simulink model "Powertrain"  (R2018b)
settings: configuration reference "Physics" (kept outside this file)
model workspace (MAT data in the model file):
  m = 1000
undefined symbols (not defined in the file): POWTR__CLUTCH__clutch_time_s, POWTR__CLUTCH__T_max_cap_Nm, POWTR__DIFFERENTIAL__c_diff_efficiency, POWTR__DIFFERENTIAL__c_diff_ratio, POWTR__DIFFERENTIAL__f_diff_efficiency, POWTR__DIFFERENTIAL__f_diff_ratio, POWTR__DIFFERENTIAL__I_drivetrain_kgm2, POWTR__DIFFERENTIAL__r_diff_efficiency, POWTR__DIFFERENTIAL__r_diff_ratio, POWTR__ENGINE__I_engine_kgm2, POWTR__ENGINE__n_0_rpm, POWTR__ENGINE__n_idle_rpm, POWTR__ENGINE__n_lb_rpm__1, POWTR__ENGINE__n_lb_rpm__2, POWTR__ENGINE__n_lb_rpm__3, POWTR__ENGINE__n_lb_rpm__4, POWTR__ENGINE__n_lb_rpm__5, POWTR__ENGINE__n_lb_rpm__6, POWTR__ENGINE__n_lb_rpm__7, POWTR__ENGINE__n_limit_rpm, POWTR__ENGINE__n_ub_rpm, POWTR__LAYOUT__p_torque_rear, POWTR__MODE__activate_CombustionEngine, POWTR__MODE__activate_ManualGearbox, POWTR__MODE__activate_ThrottleInterface, POWTR__TRANSMISSION__gear__1, POWTR__TRANSMISSION__gear__2, POWTR__TRANSMISSION__gear__3, POWTR__TRANSMISSION__gear__4, POWTR__TRANSMISSION__gear__5, POWTR__TRANSMISSION__gear__6, POWTR__TRANSMISSION__gear__7, POWTR__TRANSMISSION__gear_efficiency__1, POWTR__TRANSMISSION__gear_efficiency__2, POWTR__TRANSMISSION__gear_efficiency__3, POWTR__TRANSMISSION__gear_efficiency__4, POWTR__TRANSMISSION__gear_efficiency__5, POWTR__TRANSMISSION__gear_efficiency__6, POWTR__TRANSMISSION__gear_efficiency__7, POWTR__TRANSMISSION__gear_ratio__1, POWTR__TRANSMISSION__gear_ratio__2, POWTR__TRANSMISSION__gear_ratio__3, POWTR__TRANSMISSION__gear_ratio__4, POWTR__TRANSMISSION__gear_ratio__5, POWTR__TRANSMISSION__gear_ratio__6, POWTR__TRANSMISSION__gear_ratio__7, POWTR__TRANSMISSION__I_transmission_kgm2, tireFL__MFSIMPLE__r_tire_m, tireFR__MFSIMPLE__r_tire_m, tireRL__MFSIMPLE__r_tire_m, tireRR__MFSIMPLE__r_tire_m, VEH__VehicleData__l_WheelbaseF_m, VEH__VehicleData__l_WheelbaseTotal_m, VEH__VehicleData__w_TrackF_m, VEH__VehicleData__w_TrackR_m
libraries: simulink x4
settings Model: DataDictionary=vehicleparameters_vehdynsim.sldd  PauseTimes=9.280  Creator=wischnewski  LastModifiedBy=ga25xiw

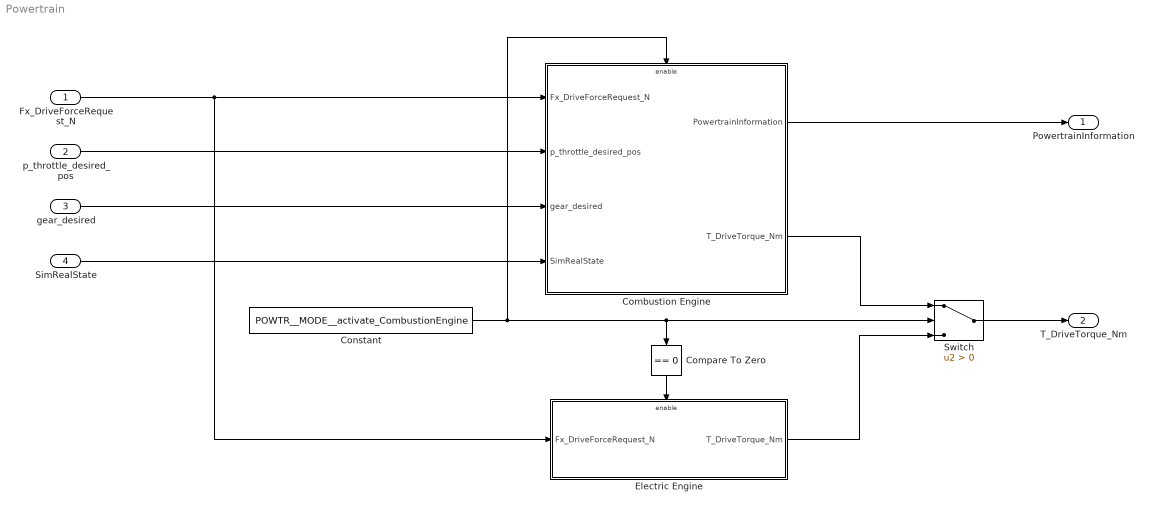
== system Powertrain ==
  Fx_DriveForceRequest_N : Inport
  p_throttle_desired_pos : Inport  Port=2
  gear_desired : Inport  Port=3
  SimRealState : Inport  Port=4  OutDataTypeStr=Bus: SimRealState
  Combustion Engine : Subsystem  TreatAsAtomicUnit=on
  Compare To Zero : simulink/Logic and Bit Operations/Compare To Zero  relop===  OutDataTypeStr=boolean
  Constant : Constant  Value=POWTR__MODE__activate_CombustionEngine
  Electric Engine : Subsystem  TreatAsAtomicUnit=on
  Switch : Switch  Criteria=u2 > Threshold
  PowertrainInformation : Outport  OutDataTypeStr=Bus: PowertrainInformation
  T_DriveTorque_Nm : Outport  Port=2
  wires:
  Constant/1 -> Combustion Engine/Enable, Switch/2, Compare To Zero/1
  gear_desired/1 -> Combustion Engine/3(gear_desired)
  Fx_DriveForceRequest_N/1 -> Electric Engine/1(Fx_DriveForceRequest_N), Combustion Engine/1(Fx_DriveForceRequest_N)
  Switch/1 -> T_DriveTorque_Nm/1
  Combustion Engine/2(T_DriveTorque_Nm) -> Switch/1
  Compare To Zero/1 -> Electric Engine/Enable
  p_throttle_desired_pos/1 -> Combustion Engine/2(p_throttle_desired_pos)
  Electric Engine/1(T_DriveTorque_Nm) -> Switch/3
  SimRealState/1 -> Combustion Engine/4(SimRealState)
  Combustion Engine/1(PowertrainInformation) -> PowertrainInformation/1

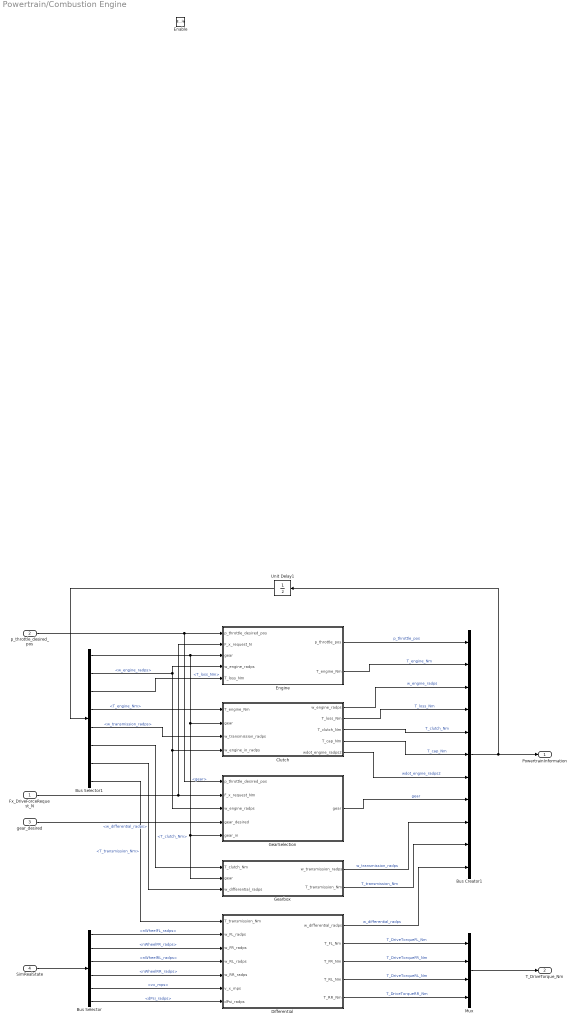
== system Powertrain/Combustion Engine ==
  Fx_DriveForceRequest_N : Inport
  p_throttle_desired_pos : Inport  Port=2
  gear_desired : Inport  Port=3
  SimRealState : Inport  Port=4  OutDataTypeStr=Bus: SimRealState
  Enable : EnablePort
  Bus Creator1 : BusCreator  Inputs=11  OutDataTypeStr=Bus: PowertrainInformation
  Bus Selector : BusSelector  OutputSignals=nWheelFL_radps,nWheelFR_radps,nWheelRL_radps,nWheelRR_radps,vx_mps,dPsi_radps
  Bus Selector1 : BusSelector  OutputSignals=gear,w_engine_radps,T_loss_Nm,T_engine_Nm,w_transmission_radps,T_clutch_Nm,w_differential_radps,T_transmission_Nm
  Clutch : Subsystem
  Differential : Subsystem
  Engine : Subsystem
  GearSelection : Subsystem
  Gearbox : Subsystem
  Mux : Mux
  Unit Delay1 : UnitDelay  SampleTime=-1
  PowertrainInformation : Outport  OutDataTypeStr=Bus: PowertrainInformation
  T_DriveTorque_Nm : Outport  Port=2
  wires:
  Differential/1(w_differential_radps) -> Bus Creator1/11  "w_differential_radps"
  Differential/4(T_RL_Nm) -> Mux/3  "T_DriveTorqueRL_Nm"
  Bus Selector1/5 -> Clutch/3(w_transmission_radps)  "<w_transmission_radps>"
  p_throttle_desired_pos/1 -> GearSelection/1(p_throttle_desired_pos), Engine/1(p_throttle_desired_pos)
  Differential/5(T_RR_Nm) -> Mux/4  "T_DriveTorqueRR_Nm"
  Engine/1(p_throttle_pos) -> Bus Creator1/1  "p_throttle_pos"
  Clutch/1(w_engine_radps) -> Bus Creator1/3  "w_engine_radps"
  Bus Creator1/1 -> Unit Delay1/1, PowertrainInformation/1
  Gearbox/1(w_transmission_radps) -> Bus Creator1/9  "w_transmission_radps"
  Mux/1 -> T_DriveTorque_Nm/1
  Bus Selector/1 -> Differential/2(w_FL_radps)  "<nWheelFL_radps>"
  Clutch/2(T_loss_Nm) -> Bus Creator1/4  "T_loss_Nm"
  Engine/2(T_engine_Nm) -> Bus Creator1/2  "T_engine_Nm"
  Fx_DriveForceRequest_N/1 -> Engine/2(F_x_request_N), GearSelection/2(F_x_request_Nm)
  Bus Selector/6 -> Differential/7(dPsi_radps)  "<dPsi_radps>"
  GearSelection/1(gear) -> Bus Creator1/8  "gear"
  Bus Selector/4 -> Differential/5(w_RR_radps)  "<nWheelRR_radps>"
  Gearbox/2(T_transmission_Nm) -> Bus Creator1/10  "T_transmission_Nm"
  SimRealState/1 -> Bus Selector/1
  Differential/2(T_FL_Nm) -> Mux/1  "T_DriveTorqueFL_Nm"
  Bus Selector/5 -> Differential/6(v_x_mps)  "<vx_mps>"
  Bus Selector1/6 -> Gearbox/1(T_clutch_Nm)  "<T_clutch_Nm>"
  Bus Selector/3 -> Differential/4(w_RL_radps)  "<nWheelRL_radps>"
  gear_desired/1 -> GearSelection/4(gear_desired)
  Differential/3(T_FR_Nm) -> Mux/2  "T_DriveTorqueFR_Nm"
  Clutch/3(T_clutch_Nm) -> Bus Creator1/5  "T_clutch_Nm"
  Bus Selector1/4 -> Clutch/1(T_engine_Nm)  "<T_engine_Nm>"
  Bus Selector1/2 -> Engine/4(w_engine_radps), GearSelection/3(w_engine_radps), Clutch/4(w_engine_in_radps)  "<w_engine_radps>"
  Bus Selector/2 -> Differential/3(w_FR_radps)  "<nWheelFR_radps>"
  Bus Selector1/7 -> Gearbox/3(w_differential_radps)  "<w_differential_radps>"
  Clutch/4(T_cap_Nm) -> Bus Creator1/6  "T_cap_Nm"
  Clutch/5(wdot_engine_radps2) -> Bus Creator1/7  "wdot_engine_radps2"
  Bus Selector1/3 -> Engine/5(T_loss_Nm)  "<T_loss_Nm>"
  Bus Selector1/1 -> Engine/3(gear), Gearbox/2(gear), GearSelection/5(gear_in), Clutch/2(gear)  "<gear>"
  Bus Selector1/8 -> Differential/1(T_transmission_Nm)  "<T_transmission_Nm>"
  Unit Delay1/1 -> Bus Selector1/1

== system Powertrain/Electric Engine ==
  Fx_DriveForceRequest_N : Inport
  Enable : EnablePort
  Constant : Constant  Value=POWTR__LAYOUT__p_torque_rear
  Demux : Demux
  EelctricEngine : MATLAB Function  TreatAsAtomicUnit=on
  Gain4 : Gain  Gain=tireFL__MFSIMPLE__r_tire_m
  Gain5 : Gain  Gain=tireFR__MFSIMPLE__r_tire_m
  Gain6 : Gain  Gain=tireRL__MFSIMPLE__r_tire_m
  Gain7 : Gain  Gain=tireRR__MFSIMPLE__r_tire_m
  Mux : Mux
  Saturation : Saturate  UpperLimit=inf  LowerLimit=0
  Transfer Fcn : TransferFcn  Denominator=[0.02 1]
  T_DriveTorque_Nm : Outport
  wires:
  EelctricEngine/1(F_DriveForce_N) -> Demux/1
  Demux/1 -> Gain4/1
  Gain6/1 -> Mux/3  "T_DriveTorqueRL_Nm"
  Constant/1 -> EelctricEngine/2(p_torque_rear)
  Saturation/1 -> Transfer Fcn/1
  Demux/3 -> Gain6/1
  Demux/2 -> Gain5/1
  Gain5/1 -> Mux/2  "T_DriveTorqueFR_Nm"
  Gain4/1 -> Mux/1  "T_DriveTorqueFL_Nm"
  Transfer Fcn/1 -> EelctricEngine/1(F_x_request_N)
  Fx_DriveForceRequest_N/1 -> Saturation/1
  Gain7/1 -> Mux/4  "T_DriveTorqueRR_Nm"
  Demux/4 -> Gain7/1
  Mux/1 -> T_DriveTorque_Nm/1

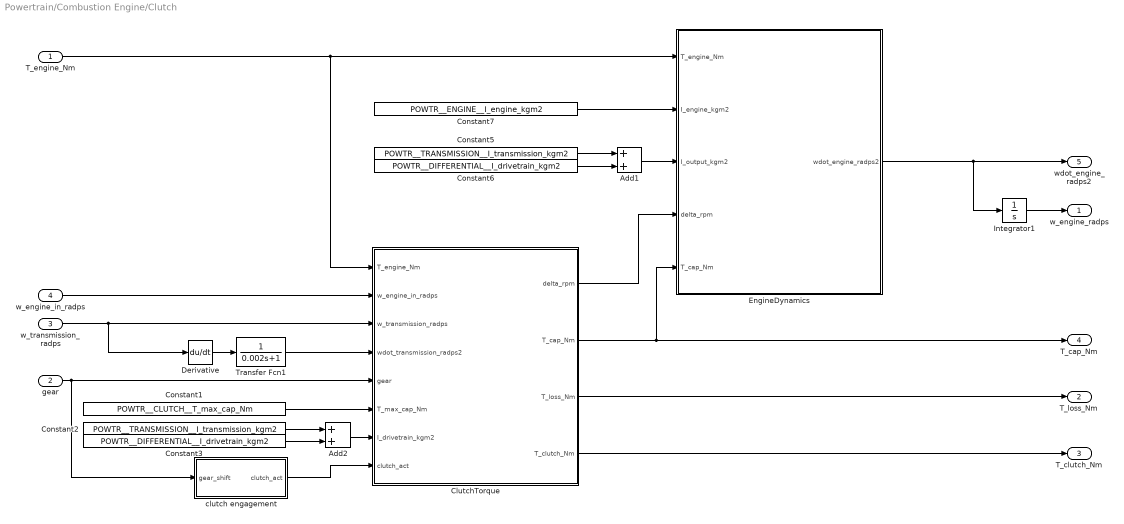
== system Powertrain/Combustion Engine/Clutch ==
  T_engine_Nm : Inport
  gear : Inport  Port=2
  w_transmission_radps : Inport  Port=3
  w_engine_in_radps : Inport  Port=4
  Add1 : Sum
  Add2 : Sum
  ClutchTorque : MATLAB Function  TreatAsAtomicUnit=on
  Constant1 : Constant  Value=POWTR__CLUTCH__T_max_cap_Nm
  Constant2 : Constant  Value=POWTR__TRANSMISSION__I_transmission_kgm2
  Constant3 : Constant  Value=POWTR__DIFFERENTIAL__I_drivetrain_kgm2
  Constant5 : Constant  Value=POWTR__TRANSMISSION__I_transmission_kgm2
  Constant6 : Constant  Value=POWTR__DIFFERENTIAL__I_drivetrain_kgm2
  Constant7 : Constant  Value=POWTR__ENGINE__I_engine_kgm2
  Derivative : Derivative
  EngineDynamics : MATLAB Function  TreatAsAtomicUnit=on
  Integrator1 : Integrator  InitialCondition=POWTR__ENGINE__n_0_rpm * ((2*pi)/60)
  Transfer Fcn1 : TransferFcn  Denominator=[0.002 1]
  clutch engagement : Subsystem
  w_engine_radps : Outport
  T_loss_Nm : Outport  Port=2
  T_clutch_Nm : Outport  Port=3
  T_cap_Nm : Outport  Port=4
  wdot_engine_radps2 : Outport  Port=5
  wires:
  ClutchTorque/1(delta_rpm) -> EngineDynamics/4(delta_rpm)
  clutch engagement/1(clutch_act) -> ClutchTorque/8(clutch_act)
  Integrator1/1 -> w_engine_radps/1
  w_transmission_radps/1 -> Derivative/1, ClutchTorque/3(w_transmission_radps)
  ClutchTorque/3(T_loss_Nm) -> T_loss_Nm/1
  ClutchTorque/2(T_cap_Nm) -> T_cap_Nm/1, EngineDynamics/5(T_cap_Nm)
  Constant7/1 -> EngineDynamics/2(I_engine_kgm2)
  ClutchTorque/4(T_clutch_Nm) -> T_clutch_Nm/1
  w_engine_in_radps/1 -> ClutchTorque/2(w_engine_in_radps)
  T_engine_Nm/1 -> ClutchTorque/1(T_engine_Nm), EngineDynamics/1(T_engine_Nm)
  Constant1/1 -> ClutchTorque/6(T_max_cap_Nm)
  Add2/1 -> ClutchTorque/7(I_drivetrain_kgm2)
  Add1/1 -> EngineDynamics/3(I_output_kgm2)
  gear/1 -> ClutchTorque/5(gear), clutch engagement/1(gear_shift)
  Constant3/1 -> Add2/2
  Transfer Fcn1/1 -> ClutchTorque/4(wdot_transmission_radps2)
  Constant2/1 -> Add2/1
  Constant5/1 -> Add1/1
  EngineDynamics/1(wdot_engine_radps2) -> Integrator1/1, wdot_engine_radps2/1
  Derivative/1 -> Transfer Fcn1/1
  Constant6/1 -> Add1/2

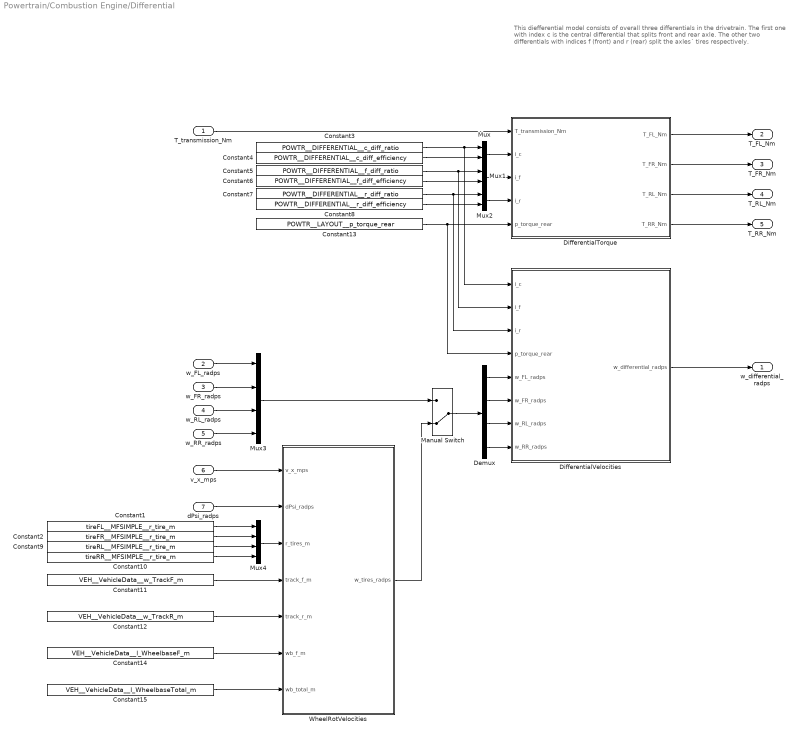
== system Powertrain/Combustion Engine/Differential ==
  note: This diefferential model consists of overall three differentials in the drivetrain.
      | The first one with index c is the central differential that splits front and rear axle.
      | The other two differentials with indices f (front) and r (rear) split the axles´ tires respectively.
  T_transmission_Nm : Inport
  w_FL_radps : Inport  Port=2
  w_FR_radps : Inport  Port=3
  w_RL_radps : Inport  Port=4
  w_RR_radps : Inport  Port=5
  v_x_mps : Inport  Port=6
  dPsi_radps : Inport  Port=7
  Constant1 : Constant  Value=tireFL__MFSIMPLE__r_tire_m
  Constant10 : Constant  Value=tireRR__MFSIMPLE__r_tire_m
  Constant11 : Constant  Value=VEH__VehicleData__w_TrackF_m
  Constant12 : Constant  Value=VEH__VehicleData__w_TrackR_m
  Constant13 : Constant  Value=POWTR__LAYOUT__p_torque_rear
  Constant14 : Constant  Value=VEH__VehicleData__l_WheelbaseF_m
  Constant15 : Constant  Value=VEH__VehicleData__l_WheelbaseTotal_m
  Constant2 : Constant  Value=tireFR__MFSIMPLE__r_tire_m
  Constant3 : Constant  Value=POWTR__DIFFERENTIAL__c_diff_ratio
  Constant4 : Constant  Value=POWTR__DIFFERENTIAL__c_diff_efficiency
  Constant5 : Constant  Value=POWTR__DIFFERENTIAL__f_diff_ratio
  Constant6 : Constant  Value=POWTR__DIFFERENTIAL__f_diff_efficiency
  Constant7 : Constant  Value=POWTR__DIFFERENTIAL__r_diff_ratio
  Constant8 : Constant  Value=POWTR__DIFFERENTIAL__r_diff_efficiency
  Constant9 : Constant  Value=tireRL__MFSIMPLE__r_tire_m
  Demux : Demux
  DifferentialTorque : MATLAB Function  TreatAsAtomicUnit=on
  DifferentialVelocities : MATLAB Function  TreatAsAtomicUnit=on
  Manual Switch : ManualSwitch  CurrentSetting=0
  Mux : Mux  Inputs=2
  Mux1 : Mux  Inputs=2
  Mux2 : Mux  Inputs=2
  Mux3 : Mux
  Mux4 : Mux
  WheelRotVelocities : MATLAB Function  TreatAsAtomicUnit=on
  w_differential_radps : Outport
  T_FL_Nm : Outport  Port=2
  T_FR_Nm : Outport  Port=3
  T_RL_Nm : Outport  Port=4
  T_RR_Nm : Outport  Port=5
  wires:
  DifferentialTorque/4(T_RR_Nm) -> T_RR_Nm/1
  Constant8/1 -> Mux2/2
  Constant11/1 -> WheelRotVelocities/4(track_f_m)
  Manual Switch/1 -> Demux/1
  Demux/1 -> DifferentialVelocities/5(w_FL_radps)
  Constant15/1 -> WheelRotVelocities/7(wb_total_m)
  Demux/4 -> DifferentialVelocities/8(w_RR_radps)
  Constant9/1 -> Mux4/3
  Mux4/1 -> WheelRotVelocities/3(r_tires_m)
  Constant14/1 -> WheelRotVelocities/6(wb_f_m)
  WheelRotVelocities/1(w_tires_radps) -> Manual Switch/2
  v_x_mps/1 -> WheelRotVelocities/1(v_x_mps)
  Constant10/1 -> Mux4/4
  Constant1/1 -> Mux4/1
  w_FL_radps/1 -> Mux3/1
  Demux/2 -> DifferentialVelocities/6(w_FR_radps)
  Constant6/1 -> Mux1/2
  w_RR_radps/1 -> Mux3/4
  dPsi_radps/1 -> WheelRotVelocities/2(dPsi_radps)
  Mux3/1 -> Manual Switch/1
  w_RL_radps/1 -> Mux3/3
  Demux/3 -> DifferentialVelocities/7(w_RL_radps)
  DifferentialTorque/3(T_RL_Nm) -> T_RL_Nm/1
  w_FR_radps/1 -> Mux3/2
  T_transmission_Nm/1 -> DifferentialTorque/1(T_transmission_Nm)
  Mux/1 -> DifferentialTorque/2(i_c)
  Constant3/1 -> Mux/1, DifferentialVelocities/1(i_c)
  Constant12/1 -> WheelRotVelocities/5(track_r_m)
  Constant4/1 -> Mux/2
  Mux2/1 -> DifferentialTorque/4(i_r)
  Constant13/1 -> DifferentialTorque/5(p_torque_rear), DifferentialVelocities/4(p_torque_rear)
  Constant5/1 -> Mux1/1, DifferentialVelocities/2(i_f)
  Constant2/1 -> Mux4/2
  DifferentialTorque/1(T_FL_Nm) -> T_FL_Nm/1
  DifferentialVelocities/1(w_differential_radps) -> w_differential_radps/1
  Mux1/1 -> DifferentialTorque/3(i_f)
  DifferentialTorque/2(T_FR_Nm) -> T_FR_Nm/1
  Constant7/1 -> Mux2/1, DifferentialVelocities/3(i_r)

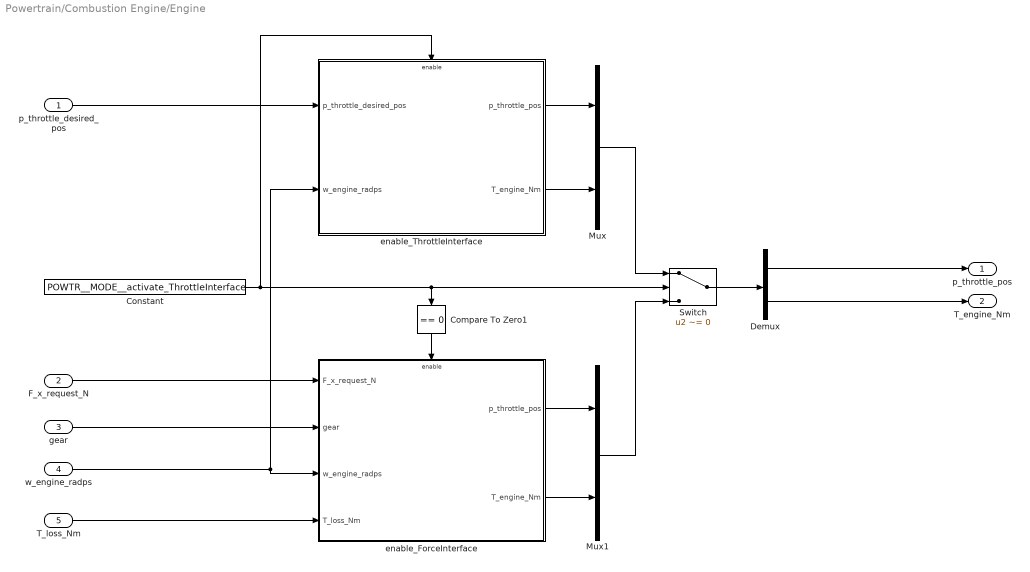
== system Powertrain/Combustion Engine/Engine ==
  p_throttle_desired_pos : Inport
  F_x_request_N : Inport  Port=2
  gear : Inport  Port=3
  w_engine_radps : Inport  Port=4
  T_loss_Nm : Inport  Port=5
  Compare To Zero1 : simulink/Logic and Bit Operations/Compare To Zero  relop===  OutDataTypeStr=uint8
  Constant : Constant  Value=POWTR__MODE__activate_ThrottleInterface
  Demux : Demux  Outputs=2
  Mux : Mux  Inputs=2
  Mux1 : Mux  Inputs=2
  Switch : Switch  Criteria=u2 ~= 0
  enable_ForceInterface : Subsystem
  enable_ThrottleInterface : Subsystem
  p_throttle_pos : Outport
  T_engine_Nm : Outport  Port=2
  wires:
  Switch/1 -> Demux/1
  Mux1/1 -> Switch/3
  Compare To Zero1/1 -> enable_ForceInterface/Enable
  T_loss_Nm/1 -> enable_ForceInterface/4(T_loss_Nm)
  gear/1 -> enable_ForceInterface/2(gear)
  w_engine_radps/1 -> enable_ForceInterface/3(w_engine_radps), enable_ThrottleInterface/2(w_engine_radps)
  enable_ForceInterface/2(T_engine_Nm) -> Mux1/2
  Constant/1 -> Switch/2, Compare To Zero1/1, enable_ThrottleInterface/Enable
  enable_ForceInterface/1(p_throttle_pos) -> Mux1/1
  F_x_request_N/1 -> enable_ForceInterface/1(F_x_request_N)
  p_throttle_desired_pos/1 -> enable_ThrottleInterface/1(p_throttle_desired_pos)
  enable_ThrottleInterface/2(T_engine_Nm) -> Mux/2
  Mux/1 -> Switch/1
  enable_ThrottleInterface/1(p_throttle_pos) -> Mux/1
  Demux/2 -> T_engine_Nm/1
  Demux/1 -> p_throttle_pos/1

== system Powertrain/Combustion Engine/GearSelection ==
  p_throttle_desired_pos : Inport
  F_x_request_Nm : Inport  Port=2
  w_engine_radps : Inport  Port=3
  gear_desired : Inport  Port=4
  gear_in : Inport  Port=5
  Compare To Zero : simulink/Logic and Bit Operations/Compare To Zero  relop===  OutDataTypeStr=boolean
  Constant1 : Constant  Value=POWTR__MODE__activate_ManualGearbox
  Switch : Switch  Criteria=u2 > Threshold
  enable_AutomaticGearbox : Subsystem
  enable_ManualGearbox : Subsystem
  gear : Outport
  wires:
  F_x_request_Nm/1 -> enable_AutomaticGearbox/2(F_x_request_Nm)
  p_throttle_desired_pos/1 -> enable_AutomaticGearbox/1(p_throttle_desired_pos)
  Compare To Zero/1 -> enable_AutomaticGearbox/Enable
  enable_ManualGearbox/1(gear) -> Switch/1
  Switch/1 -> gear/1
  Constant1/1 -> Switch/2, Compare To Zero/1, enable_ManualGearbox/Enable
  gear_in/1 -> enable_AutomaticGearbox/4(gear_in), enable_ManualGearbox/2(gear_in)
  enable_AutomaticGearbox/1(gear) -> Switch/3
  gear_desired/1 -> enable_ManualGearbox/3(gear_desired)
  w_engine_radps/1 -> enable_AutomaticGearbox/3(w_engine_radps), enable_ManualGearbox/1(w_engine_radps)

== system Powertrain/Combustion Engine/Gearbox ==
  T_clutch_Nm : Inport
  gear : Inport  Port=2
  w_differential_radps : Inport  Port=3
  Subsystem : Subsystem
  Transfer Fcn1 : TransferFcn  Denominator=[0.05 1]
  Transfer Fcn2 : TransferFcn  Denominator=[0.002 1]
  TransmissionTorque : MATLAB Function  TreatAsAtomicUnit=on
  TransmissionVelocity : MATLAB Function  TreatAsAtomicUnit=on
  w_transmission_radps : Outport
  T_transmission_Nm : Outport  Port=2
  wires:
  TransmissionVelocity/1(w_transmission_radps) -> Transfer Fcn2/1
  TransmissionTorque/1(T_transmission_Nm) -> Transfer Fcn1/1
  w_differential_radps/1 -> TransmissionVelocity/3(w_diff_radps)
  Transfer Fcn1/1 -> T_transmission_Nm/1
  T_clutch_Nm/1 -> TransmissionTorque/1(T_clutch_Nm)
  Subsystem/1(i_gearset) -> TransmissionTorque/3(i_gearset), TransmissionVelocity/1(i_gearset)
  gear/1 -> TransmissionTorque/2(gear), TransmissionVelocity/2(gear)
  Transfer Fcn2/1 -> w_transmission_radps/1

== system Powertrain/Combustion Engine/Clutch/clutch engagement ==
  gear_shift : Inport
  Constant : Constant  Value=0.25
  Constant4 : Constant  Value=POWTR__CLUTCH__clutch_time_s
  Derivative1 : Derivative
  Divide : Product  Inputs=*/
  Integrator : Integrator  ExternalReset=level hold
  Saturation : Saturate  UpperLimit=1  LowerLimit=0
  clutch_act : Outport
  wires:
  gear_shift/1 -> Derivative1/1
  Divide/1 -> Integrator/1
  Constant4/1 -> Divide/2
  Derivative1/1 -> Integrator/2
  Constant/1 -> Divide/1
  Integrator/1 -> Saturation/1
  Saturation/1 -> clutch_act/1

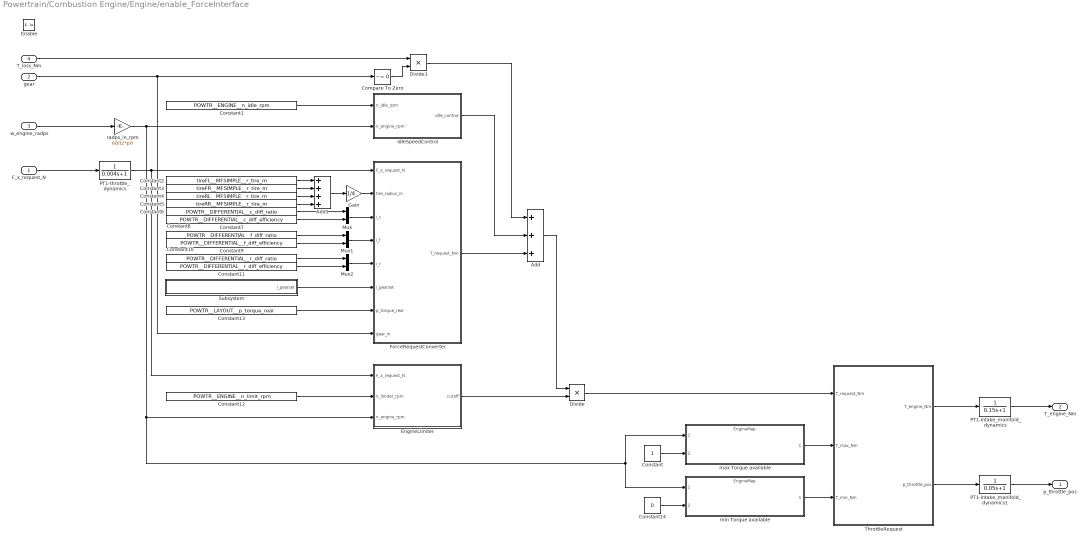
== system Powertrain/Combustion Engine/Engine/enable_ForceInterface ==
  F_x_request_N : Inport
  gear : Inport  Port=2
  w_engine_radps : Inport  Port=3
  T_loss_Nm : Inport  Port=4
  Enable : EnablePort
  Add : Sum  Inputs=+++
  Add1 : Sum  Inputs=++++
  Compare To Zero : simulink/Logic and Bit Operations/Compare To Zero  relop=~=  OutDataTypeStr=boolean
  Constant : Constant
  Constant1 : Constant  Value=POWTR__ENGINE__n_idle_rpm
  Constant10 : Constant  Value=POWTR__DIFFERENTIAL__r_diff_ratio
  Constant11 : Constant  Value=POWTR__DIFFERENTIAL__r_diff_efficiency
  Constant12 : Constant  Value=POWTR__ENGINE__n_limit_rpm
  Constant13 : Constant  Value=POWTR__LAYOUT__p_torque_rear
  Constant14 : Constant  Value=0
  Constant2 : Constant  Value=tireFL__MFSIMPLE__r_tire_m
  Constant3 : Constant  Value=tireFR__MFSIMPLE__r_tire_m
  Constant4 : Constant  Value=tireRL__MFSIMPLE__r_tire_m
  Constant5 : Constant  Value=tireRR__MFSIMPLE__r_tire_m
  Constant6 : Constant  Value=POWTR__DIFFERENTIAL__c_diff_ratio
  Constant7 : Constant  Value=POWTR__DIFFERENTIAL__c_diff_efficiency
  Constant8 : Constant  Value=POWTR__DIFFERENTIAL__f_diff_ratio
  Constant9 : Constant  Value=POWTR__DIFFERENTIAL__f_diff_efficiency
  Divide : Product  Inputs=**
  Divide1 : Product  Inputs=**
  EngineLimiter : MATLAB Function  TreatAsAtomicUnit=on
  ForceRequestConverter : MATLAB Function  TreatAsAtomicUnit=on
  Gain : Gain  Gain=1/4
  IdleSpeedControl : MATLAB Function  TreatAsAtomicUnit=on
  Mux : Mux  Inputs=2
  Mux1 : Mux  Inputs=2
  Mux2 : Mux  Inputs=2
  PT1-intake_manifold_dynamics : TransferFcn  Denominator=[0.15 1]
  PT1-intake_manifold_dynamics1 : TransferFcn  Denominator=[0.05 1]
  PT1-throttle_dynamics : TransferFcn  Denominator=[0.004 1]
  Subsystem : Subsystem
  ThrottleRequest : MATLAB Function  TreatAsAtomicUnit=on
  max Torque available : ModelReference  ModelNameDialog=EngineMap.slx  SimulationMode=Normal  ModelReferenceVersion=1.393
  min Torque available : ModelReference  ModelNameDialog=EngineMap.slx  SimulationMode=Normal  ModelReferenceVersion=1.393
  radps_in_rpm : Gain  Gain=60/(2*pi)
  p_throttle_pos : Outport
  T_engine_Nm : Outport  Port=2
  wires:
  Constant8/1 -> Mux1/1
  gear/1 -> Compare To Zero/1, ForceRequestConverter/8(gear_in)
  PT1-throttle_dynamics/1 -> ForceRequestConverter/1(F_x_request_N), EngineLimiter/1(F_x_request_N)
  Constant5/1 -> Add1/4
  Constant13/1 -> ForceRequestConverter/7(p_torque_rear)
  Constant7/1 -> Mux/2
  Compare To Zero/1 -> Divide1/2
  T_loss_Nm/1 -> Divide1/1
  EngineLimiter/1(cutoff) -> Divide/2
  Constant3/1 -> Add1/2
  Constant12/1 -> EngineLimiter/2(n_limiter_rpm)
  ForceRequestConverter/1(T_request_Nm) -> Add/3
  Add1/1 -> Gain/1
  IdleSpeedControl/1(idle_control) -> Add/2
  PT1-intake_manifold_dynamics1/1 -> p_throttle_pos/1
  Constant4/1 -> Add1/3
  Mux2/1 -> ForceRequestConverter/5(i_r)
  Divide1/1 -> Add/1
  Constant11/1 -> Mux2/2
  ThrottleRequest/1(T_engine_Nm) -> PT1-intake_manifold_dynamics/1
  Constant10/1 -> Mux2/1
  Mux/1 -> ForceRequestConverter/3(i_c)
  Constant2/1 -> Add1/1
  ThrottleRequest/2(p_throttle_pos) -> PT1-intake_manifold_dynamics1/1
  Mux1/1 -> ForceRequestConverter/4(i_f)
  PT1-intake_manifold_dynamics/1 -> T_engine_Nm/1
  F_x_request_N/1 -> PT1-throttle_dynamics/1
  Add/1 -> Divide/1
  Subsystem/1(i_gearset) -> ForceRequestConverter/6(i_gearset)
  Constant9/1 -> Mux1/2
  w_engine_radps/1 -> radps_in_rpm/1
  Constant1/1 -> IdleSpeedControl/1(n_idle_rpm)
  Gain/1 -> ForceRequestConverter/2(tire_radius_m)
  Constant6/1 -> Mux/1
  Constant14/1 -> min Torque available/2
  radps_in_rpm/1 -> IdleSpeedControl/2(n_engine_rpm), EngineLimiter/3(n_engine_rpm), min Torque available/1, max Torque available/1
  min Torque available/1 -> ThrottleRequest/3(T_min_Nm)
  Divide/1 -> ThrottleRequest/1(T_request_Nm)
  max Torque available/1 -> ThrottleRequest/2(T_max_Nm)
  Constant/1 -> max Torque available/2

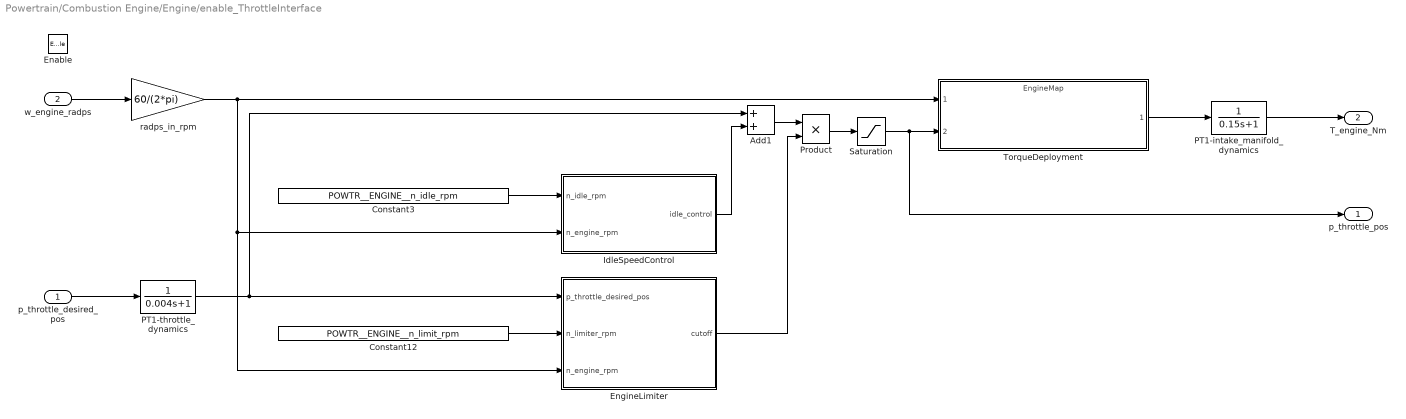
== system Powertrain/Combustion Engine/Engine/enable_ThrottleInterface ==
  p_throttle_desired_pos : Inport
  w_engine_radps : Inport  Port=2
  Enable : EnablePort
  Add1 : Sum
  Constant12 : Constant  Value=POWTR__ENGINE__n_limit_rpm
  Constant3 : Constant  Value=POWTR__ENGINE__n_idle_rpm
  EngineLimiter : MATLAB Function  TreatAsAtomicUnit=on
  IdleSpeedControl : MATLAB Function  TreatAsAtomicUnit=on
  PT1-intake_manifold_dynamics : TransferFcn  Denominator=[0.15 1]
  PT1-throttle_dynamics : TransferFcn  Denominator=[0.004 1]
  Product : Product
  Saturation : Saturate  UpperLimit=1  LowerLimit=0
  TorqueDeployment : ModelReference  ModelNameDialog=EngineMap.slx  SimulationMode=Normal  ModelReferenceVersion=1.393
  radps_in_rpm : Gain  Gain=60/(2*pi)
  p_throttle_pos : Outport
  T_engine_Nm : Outport  Port=2
  wires:
  Constant12/1 -> EngineLimiter/2(n_limiter_rpm)
  Product/1 -> Saturation/1
  Add1/1 -> Product/1
  EngineLimiter/1(cutoff) -> Product/2
  IdleSpeedControl/1(idle_control) -> Add1/2
  w_engine_radps/1 -> radps_in_rpm/1
  p_throttle_desired_pos/1 -> PT1-throttle_dynamics/1
  Saturation/1 -> TorqueDeployment/2, p_throttle_pos/1
  PT1-intake_manifold_dynamics/1 -> T_engine_Nm/1
  TorqueDeployment/1 -> PT1-intake_manifold_dynamics/1
  radps_in_rpm/1 -> EngineLimiter/3(n_engine_rpm), IdleSpeedControl/2(n_engine_rpm), TorqueDeployment/1
  PT1-throttle_dynamics/1 -> Add1/1, EngineLimiter/1(p_throttle_desired_pos)
  Constant3/1 -> IdleSpeedControl/1(n_idle_rpm)

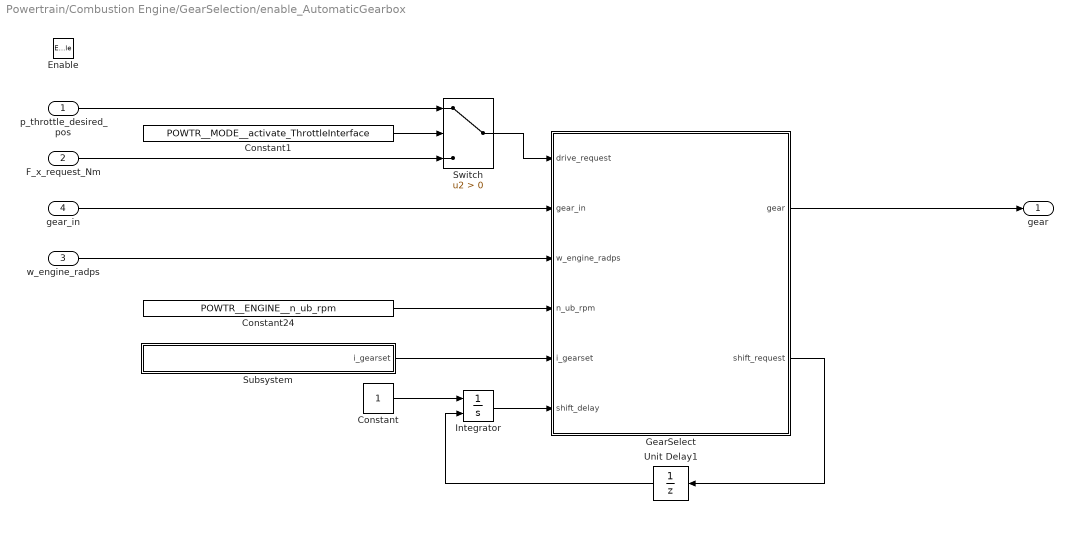
== system Powertrain/Combustion Engine/GearSelection/enable_AutomaticGearbox ==
  p_throttle_desired_pos : Inport
  F_x_request_Nm : Inport  Port=2
  w_engine_radps : Inport  Port=3
  gear_in : Inport  Port=4
  Enable : EnablePort
  Constant : Constant
  Constant1 : Constant  Value=POWTR__MODE__activate_ThrottleInterface
  Constant24 : Constant  Value=POWTR__ENGINE__n_ub_rpm
  GearSelect : MATLAB Function  TreatAsAtomicUnit=on
  Integrator : Integrator  ExternalReset=rising
  Subsystem : Subsystem
  Switch : Switch  Criteria=u2 > Threshold
  Unit Delay1 : UnitDelay  SampleTime=-1
  gear : Outport
  wires:
  GearSelect/1(gear) -> gear/1
  gear_in/1 -> GearSelect/2(gear_in)
  Constant1/1 -> Switch/2
  Integrator/1 -> GearSelect/6(shift_delay)
  p_throttle_desired_pos/1 -> Switch/1
  w_engine_radps/1 -> GearSelect/3(w_engine_radps)
  Subsystem/1(i_gearset) -> GearSelect/5(i_gearset)
  Unit Delay1/1 -> Integrator/2
  Constant24/1 -> GearSelect/4(n_ub_rpm)
  Constant/1 -> Integrator/1
  Switch/1 -> GearSelect/1(drive_request)
  GearSelect/2(shift_request) -> Unit Delay1/1
  F_x_request_Nm/1 -> Switch/3

== system Powertrain/Combustion Engine/GearSelection/enable_ManualGearbox ==
  w_engine_radps : Inport
  gear_in : Inport  Port=2
  gear_desired : Inport  Port=3
  Enable : EnablePort
  Constant : Constant
  Integrator : Integrator  ExternalReset=rising
  ManualGearbox : MATLAB Function  TreatAsAtomicUnit=on
  Subsystem : Subsystem
  Unit Delay1 : UnitDelay  SampleTime=-1
  gear : Outport
  wires:
  ManualGearbox/2(shift_request) -> Unit Delay1/1
  Constant/1 -> Integrator/1
  Unit Delay1/1 -> Integrator/2
  Subsystem/1(i_gearset) -> ManualGearbox/4(i_gearset)
  w_engine_radps/1 -> ManualGearbox/3(w_engine_radps)
  Integrator/1 -> ManualGearbox/5(shift_delay)
  gear_in/1 -> ManualGearbox/1(gear_in)
  ManualGearbox/1(gear) -> gear/1
  gear_desired/1 -> ManualGearbox/2(gear_desired)

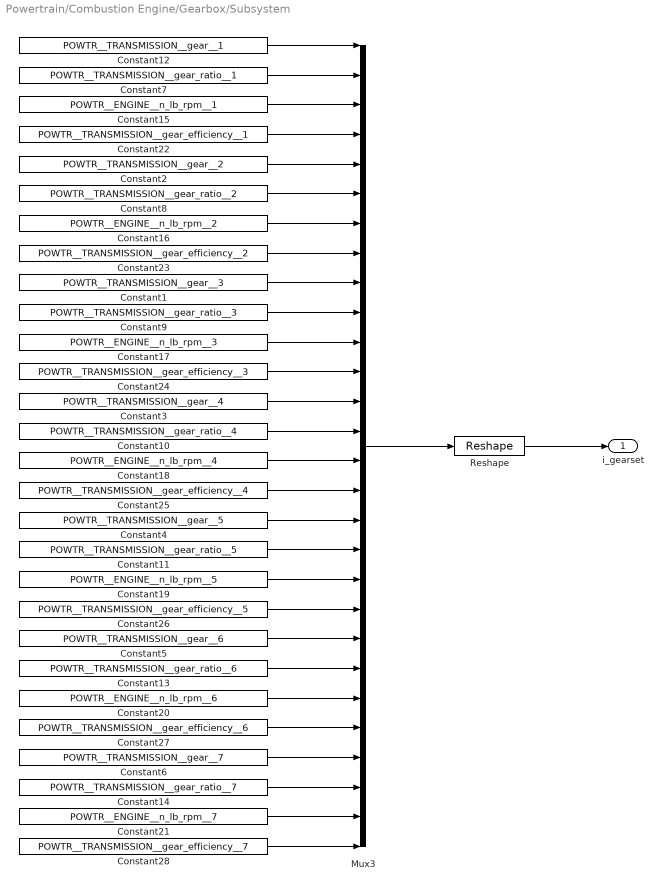
== system Powertrain/Combustion Engine/Gearbox/Subsystem ==
  Constant1 : Constant  Value=POWTR__TRANSMISSION__gear__3
  Constant10 : Constant  Value=POWTR__TRANSMISSION__gear_ratio__4
  Constant11 : Constant  Value=POWTR__TRANSMISSION__gear_ratio__5
  Constant12 : Constant  Value=POWTR__TRANSMISSION__gear__1
  Constant13 : Constant  Value=POWTR__TRANSMISSION__gear_ratio__6
  Constant14 : Constant  Value=POWTR__TRANSMISSION__gear_ratio__7
  Constant15 : Constant  Value=POWTR__ENGINE__n_lb_rpm__1
  Constant16 : Constant  Value=POWTR__ENGINE__n_lb_rpm__2
  Constant17 : Constant  Value=POWTR__ENGINE__n_lb_rpm__3
  Constant18 : Constant  Value=POWTR__ENGINE__n_lb_rpm__4
  Constant19 : Constant  Value=POWTR__ENGINE__n_lb_rpm__5
  Constant2 : Constant  Value=POWTR__TRANSMISSION__gear__2
  Constant20 : Constant  Value=POWTR__ENGINE__n_lb_rpm__6
  Constant21 : Constant  Value=POWTR__ENGINE__n_lb_rpm__7
  Constant22 : Constant  Value=POWTR__TRANSMISSION__gear_efficiency__1
  Constant23 : Constant  Value=POWTR__TRANSMISSION__gear_efficiency__2
  Constant24 : Constant  Value=POWTR__TRANSMISSION__gear_efficiency__3
  Constant25 : Constant  Value=POWTR__TRANSMISSION__gear_efficiency__4
  Constant26 : Constant  Value=POWTR__TRANSMISSION__gear_efficiency__5
  Constant27 : Constant  Value=POWTR__TRANSMISSION__gear_efficiency__6
  Constant28 : Constant  Value=POWTR__TRANSMISSION__gear_efficiency__7
  Constant3 : Constant  Value=POWTR__TRANSMISSION__gear__4
  Constant4 : Constant  Value=POWTR__TRANSMISSION__gear__5
  Constant5 : Constant  Value=POWTR__TRANSMISSION__gear__6
  Constant6 : Constant  Value=POWTR__TRANSMISSION__gear__7
  Constant7 : Constant  Value=POWTR__TRANSMISSION__gear_ratio__1
  Constant8 : Constant  Value=POWTR__TRANSMISSION__gear_ratio__2
  Constant9 : Constant  Value=POWTR__TRANSMISSION__gear_ratio__3
  Mux3 : Mux  Inputs=28
  Reshape : Reshape  OutputDimensionality=Customize  OutputDimensions=[4,7]
  i_gearset : Outport
  wires:
  Mux3/1 -> Reshape/1
  Constant12/1 -> Mux3/1
  Reshape/1 -> i_gearset/1
  Constant2/1 -> Mux3/5
  Constant1/1 -> Mux3/9
  Constant3/1 -> Mux3/13
  Constant4/1 -> Mux3/17
  Constant5/1 -> Mux3/21
  Constant6/1 -> Mux3/25
  Constant7/1 -> Mux3/2
  Constant8/1 -> Mux3/6
  Constant9/1 -> Mux3/10
  Constant10/1 -> Mux3/14
  Constant11/1 -> Mux3/18
  Constant13/1 -> Mux3/22
  Constant14/1 -> Mux3/26
  Constant15/1 -> Mux3/3
  Constant16/1 -> Mux3/7
  Constant17/1 -> Mux3/11
  Constant18/1 -> Mux3/15
  Constant19/1 -> Mux3/19
  Constant20/1 -> Mux3/23
  Constant21/1 -> Mux3/27
  Constant22/1 -> Mux3/4
  Constant23/1 -> Mux3/8
  Constant24/1 -> Mux3/12
  Constant25/1 -> Mux3/16
  Constant26/1 -> Mux3/20
  Constant27/1 -> Mux3/24
  Constant28/1 -> Mux3/28

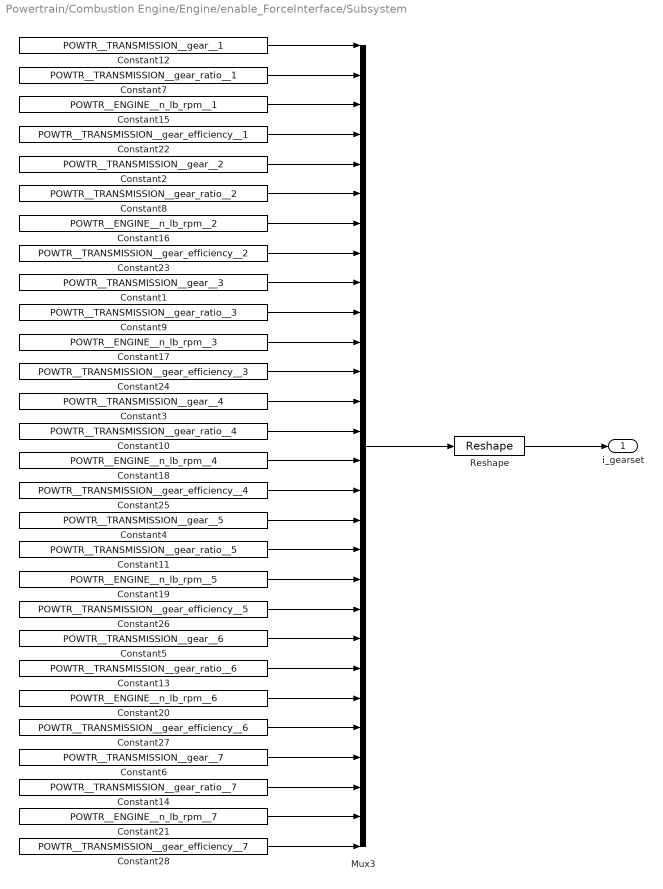
== system Powertrain/Combustion Engine/Engine/enable_ForceInterface/Subsystem ==
  Constant1 : Constant  Value=POWTR__TRANSMISSION__gear__3
  Constant10 : Constant  Value=POWTR__TRANSMISSION__gear_ratio__4
  Constant11 : Constant  Value=POWTR__TRANSMISSION__gear_ratio__5
  Constant12 : Constant  Value=POWTR__TRANSMISSION__gear__1
  Constant13 : Constant  Value=POWTR__TRANSMISSION__gear_ratio__6
  Constant14 : Constant  Value=POWTR__TRANSMISSION__gear_ratio__7
  Constant15 : Constant  Value=POWTR__ENGINE__n_lb_rpm__1
  Constant16 : Constant  Value=POWTR__ENGINE__n_lb_rpm__2
  Constant17 : Constant  Value=POWTR__ENGINE__n_lb_rpm__3
  Constant18 : Constant  Value=POWTR__ENGINE__n_lb_rpm__4
  Constant19 : Constant  Value=POWTR__ENGINE__n_lb_rpm__5
  Constant2 : Constant  Value=POWTR__TRANSMISSION__gear__2
  Constant20 : Constant  Value=POWTR__ENGINE__n_lb_rpm__6
  Constant21 : Constant  Value=POWTR__ENGINE__n_lb_rpm__7
  Constant22 : Constant  Value=POWTR__TRANSMISSION__gear_efficiency__1
  Constant23 : Constant  Value=POWTR__TRANSMISSION__gear_efficiency__2
  Constant24 : Constant  Value=POWTR__TRANSMISSION__gear_efficiency__3
  Constant25 : Constant  Value=POWTR__TRANSMISSION__gear_efficiency__4
  Constant26 : Constant  Value=POWTR__TRANSMISSION__gear_efficiency__5
  Constant27 : Constant  Value=POWTR__TRANSMISSION__gear_efficiency__6
  Constant28 : Constant  Value=POWTR__TRANSMISSION__gear_efficiency__7
  Constant3 : Constant  Value=POWTR__TRANSMISSION__gear__4
  Constant4 : Constant  Value=POWTR__TRANSMISSION__gear__5
  Constant5 : Constant  Value=POWTR__TRANSMISSION__gear__6
  Constant6 : Constant  Value=POWTR__TRANSMISSION__gear__7
  Constant7 : Constant  Value=POWTR__TRANSMISSION__gear_ratio__1
  Constant8 : Constant  Value=POWTR__TRANSMISSION__gear_ratio__2
  Constant9 : Constant  Value=POWTR__TRANSMISSION__gear_ratio__3
  Mux3 : Mux  Inputs=28
  Reshape : Reshape  OutputDimensionality=Customize  OutputDimensions=[4,7]
  i_gearset : Outport
  wires:
  Mux3/1 -> Reshape/1
  Constant12/1 -> Mux3/1
  Reshape/1 -> i_gearset/1
  Constant2/1 -> Mux3/5
  Constant1/1 -> Mux3/9
  Constant3/1 -> Mux3/13
  Constant4/1 -> Mux3/17
  Constant5/1 -> Mux3/21
  Constant6/1 -> Mux3/25
  Constant7/1 -> Mux3/2
  Constant8/1 -> Mux3/6
  Constant9/1 -> Mux3/10
  Constant10/1 -> Mux3/14
  Constant11/1 -> Mux3/18
  Constant13/1 -> Mux3/22
  Constant14/1 -> Mux3/26
  Constant15/1 -> Mux3/3
  Constant16/1 -> Mux3/7
  Constant17/1 -> Mux3/11
  Constant18/1 -> Mux3/15
  Constant19/1 -> Mux3/19
  Constant20/1 -> Mux3/23
  Constant21/1 -> Mux3/27
  Constant22/1 -> Mux3/4
  Constant23/1 -> Mux3/8
  Constant24/1 -> Mux3/12
  Constant25/1 -> Mux3/16
  Constant26/1 -> Mux3/20
  Constant27/1 -> Mux3/24
  Constant28/1 -> Mux3/28

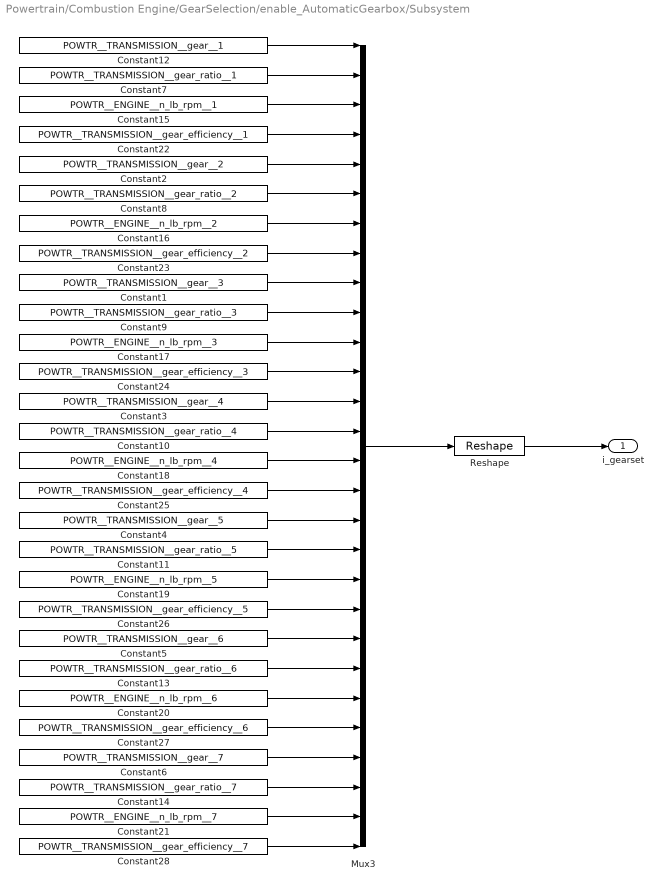
== system Powertrain/Combustion Engine/GearSelection/enable_AutomaticGearbox/Subsystem ==
  Constant1 : Constant  Value=POWTR__TRANSMISSION__gear__3
  Constant10 : Constant  Value=POWTR__TRANSMISSION__gear_ratio__4
  Constant11 : Constant  Value=POWTR__TRANSMISSION__gear_ratio__5
  Constant12 : Constant  Value=POWTR__TRANSMISSION__gear__1
  Constant13 : Constant  Value=POWTR__TRANSMISSION__gear_ratio__6
  Constant14 : Constant  Value=POWTR__TRANSMISSION__gear_ratio__7
  Constant15 : Constant  Value=POWTR__ENGINE__n_lb_rpm__1
  Constant16 : Constant  Value=POWTR__ENGINE__n_lb_rpm__2
  Constant17 : Constant  Value=POWTR__ENGINE__n_lb_rpm__3
  Constant18 : Constant  Value=POWTR__ENGINE__n_lb_rpm__4
  Constant19 : Constant  Value=POWTR__ENGINE__n_lb_rpm__5
  Constant2 : Constant  Value=POWTR__TRANSMISSION__gear__2
  Constant20 : Constant  Value=POWTR__ENGINE__n_lb_rpm__6
  Constant21 : Constant  Value=POWTR__ENGINE__n_lb_rpm__7
  Constant22 : Constant  Value=POWTR__TRANSMISSION__gear_efficiency__1
  Constant23 : Constant  Value=POWTR__TRANSMISSION__gear_efficiency__2
  Constant24 : Constant  Value=POWTR__TRANSMISSION__gear_efficiency__3
  Constant25 : Constant  Value=POWTR__TRANSMISSION__gear_efficiency__4
  Constant26 : Constant  Value=POWTR__TRANSMISSION__gear_efficiency__5
  Constant27 : Constant  Value=POWTR__TRANSMISSION__gear_efficiency__6
  Constant28 : Constant  Value=POWTR__TRANSMISSION__gear_efficiency__7
  Constant3 : Constant  Value=POWTR__TRANSMISSION__gear__4
  Constant4 : Constant  Value=POWTR__TRANSMISSION__gear__5
  Constant5 : Constant  Value=POWTR__TRANSMISSION__gear__6
  Constant6 : Constant  Value=POWTR__TRANSMISSION__gear__7
  Constant7 : Constant  Value=POWTR__TRANSMISSION__gear_ratio__1
  Constant8 : Constant  Value=POWTR__TRANSMISSION__gear_ratio__2
  Constant9 : Constant  Value=POWTR__TRANSMISSION__gear_ratio__3
  Mux3 : Mux  Inputs=28
  Reshape : Reshape  OutputDimensionality=Customize  OutputDimensions=[4,7]
  i_gearset : Outport
  wires:
  Mux3/1 -> Reshape/1
  Constant12/1 -> Mux3/1
  Reshape/1 -> i_gearset/1
  Constant2/1 -> Mux3/5
  Constant1/1 -> Mux3/9
  Constant3/1 -> Mux3/13
  Constant4/1 -> Mux3/17
  Constant5/1 -> Mux3/21
  Constant6/1 -> Mux3/25
  Constant7/1 -> Mux3/2
  Constant8/1 -> Mux3/6
  Constant9/1 -> Mux3/10
  Constant10/1 -> Mux3/14
  Constant11/1 -> Mux3/18
  Constant13/1 -> Mux3/22
  Constant14/1 -> Mux3/26
  Constant15/1 -> Mux3/3
  Constant16/1 -> Mux3/7
  Constant17/1 -> Mux3/11
  Constant18/1 -> Mux3/15
  Constant19/1 -> Mux3/19
  Constant20/1 -> Mux3/23
  Constant21/1 -> Mux3/27
  Constant22/1 -> Mux3/4
  Constant23/1 -> Mux3/8
  Constant24/1 -> Mux3/12
  Constant25/1 -> Mux3/16
  Constant26/1 -> Mux3/20
  Constant27/1 -> Mux3/24
  Constant28/1 -> Mux3/28

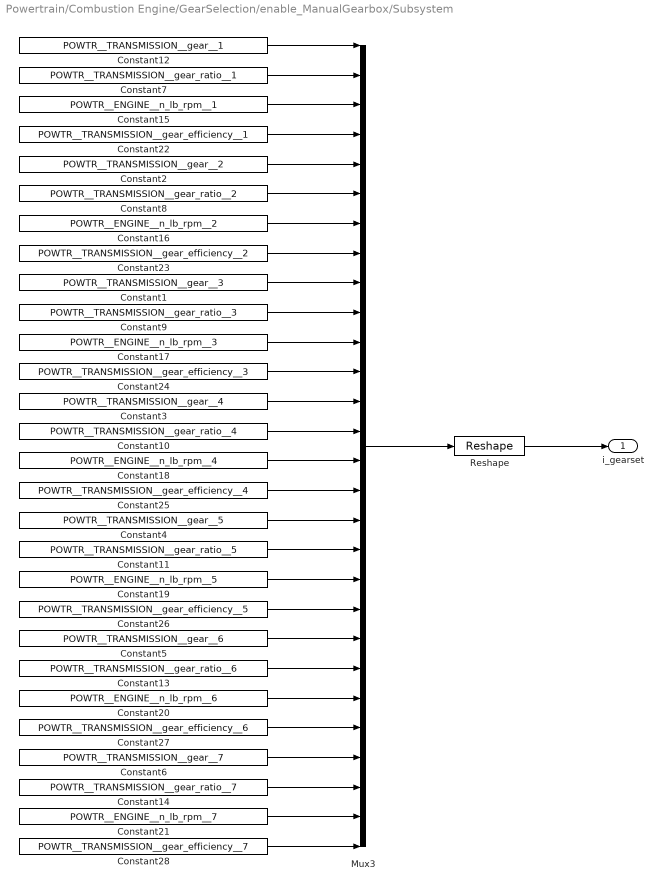
== system Powertrain/Combustion Engine/GearSelection/enable_ManualGearbox/Subsystem ==
  Constant1 : Constant  Value=POWTR__TRANSMISSION__gear__3
  Constant10 : Constant  Value=POWTR__TRANSMISSION__gear_ratio__4
  Constant11 : Constant  Value=POWTR__TRANSMISSION__gear_ratio__5
  Constant12 : Constant  Value=POWTR__TRANSMISSION__gear__1
  Constant13 : Constant  Value=POWTR__TRANSMISSION__gear_ratio__6
  Constant14 : Constant  Value=POWTR__TRANSMISSION__gear_ratio__7
  Constant15 : Constant  Value=POWTR__ENGINE__n_lb_rpm__1
  Constant16 : Constant  Value=POWTR__ENGINE__n_lb_rpm__2
  Constant17 : Constant  Value=POWTR__ENGINE__n_lb_rpm__3
  Constant18 : Constant  Value=POWTR__ENGINE__n_lb_rpm__4
  Constant19 : Constant  Value=POWTR__ENGINE__n_lb_rpm__5
  Constant2 : Constant  Value=POWTR__TRANSMISSION__gear__2
  Constant20 : Constant  Value=POWTR__ENGINE__n_lb_rpm__6
  Constant21 : Constant  Value=POWTR__ENGINE__n_lb_rpm__7
  Constant22 : Constant  Value=POWTR__TRANSMISSION__gear_efficiency__1
  Constant23 : Constant  Value=POWTR__TRANSMISSION__gear_efficiency__2
  Constant24 : Constant  Value=POWTR__TRANSMISSION__gear_efficiency__3
  Constant25 : Constant  Value=POWTR__TRANSMISSION__gear_efficiency__4
  Constant26 : Constant  Value=POWTR__TRANSMISSION__gear_efficiency__5
  Constant27 : Constant  Value=POWTR__TRANSMISSION__gear_efficiency__6
  Constant28 : Constant  Value=POWTR__TRANSMISSION__gear_efficiency__7
  Constant3 : Constant  Value=POWTR__TRANSMISSION__gear__4
  Constant4 : Constant  Value=POWTR__TRANSMISSION__gear__5
  Constant5 : Constant  Value=POWTR__TRANSMISSION__gear__6
  Constant6 : Constant  Value=POWTR__TRANSMISSION__gear__7
  Constant7 : Constant  Value=POWTR__TRANSMISSION__gear_ratio__1
  Constant8 : Constant  Value=POWTR__TRANSMISSION__gear_ratio__2
  Constant9 : Constant  Value=POWTR__TRANSMISSION__gear_ratio__3
  Mux3 : Mux  Inputs=28
  Reshape : Reshape  OutputDimensionality=Customize  OutputDimensions=[4,7]
  i_gearset : Outport
  wires:
  Constant28/1 -> Mux3/28
  Constant27/1 -> Mux3/24
  Constant26/1 -> Mux3/20
  Constant25/1 -> Mux3/16
  Constant24/1 -> Mux3/12
  Constant23/1 -> Mux3/8
  Constant22/1 -> Mux3/4
  Constant21/1 -> Mux3/27
  Constant20/1 -> Mux3/23
  Constant19/1 -> Mux3/19
  Constant18/1 -> Mux3/15
  Constant17/1 -> Mux3/11
  Constant16/1 -> Mux3/7
  Constant15/1 -> Mux3/3
  Constant14/1 -> Mux3/26
  Constant13/1 -> Mux3/22
  Constant11/1 -> Mux3/18
  Constant10/1 -> Mux3/14
  Constant9/1 -> Mux3/10
  Constant8/1 -> Mux3/6
  Constant7/1 -> Mux3/2
  Constant6/1 -> Mux3/25
  Constant5/1 -> Mux3/21
  Constant4/1 -> Mux3/17
  Constant3/1 -> Mux3/13
  Constant1/1 -> Mux3/9
  Constant2/1 -> Mux3/5
  Reshape/1 -> i_gearset/1
  Constant12/1 -> Mux3/1
  Mux3/1 -> Reshape/1

== matlab function Powertrain/Combustion Engine/Differential/DifferentialTorque ==
  data: T_transmission_Nm input; i_c input; T_FL_Nm output; i_f input; i_r input; p_torque_rear input; T_FR_Nm output; T_RL_Nm output; T_RR_Nm output
function [T_FL_Nm, T_FR_Nm, T_RL_Nm, T_RR_Nm] = fcn(...
                        T_transmission_Nm, i_c, i_f, i_r, p_torque_rear)

[T_FL_Nm, T_FR_Nm, T_RL_Nm, T_RR_Nm] = DifferentialTorque(...
                        T_transmission_Nm, i_c, i_f, i_r, p_torque_rear);

== matlab function Powertrain/Electric Engine/EelctricEngine ==
  data: F_x_request_N input; F_DriveForce_N output; p_torque_rear input
function F_DriveForce_N = fcn(F_x_request_N, p_torque_rear)

F_DriveForce_N = ElectricEngine(F_x_request_N, p_torque_rear);

== matlab function Powertrain/Combustion Engine/Differential/DifferentialVelocities ==
  data: i_c input; w_differential_radps output; i_f input; i_r input; p_torque_rear input; w_FL_radps input; w_FR_radps input; w_RL_radps input; w_RR_radps input
function w_differential_radps = fcn(...
                        i_c, i_f, i_r, p_torque_rear, ...
                        w_FL_radps, w_FR_radps, w_RL_radps, w_RR_radps)

w_differential_radps = DifferentialVelocities(...
                        i_c, i_f, i_r, p_torque_rear, ...
                        w_FL_radps, w_FR_radps, w_RL_radps, w_RR_radps);

== matlab function Powertrain/Combustion Engine/Differential/WheelRotVelocities ==
  data: v_x_mps input; w_tires_radps output; dPsi_radps input; r_tires_m input; track_f_m input; track_r_m input; wb_f_m input; wb_total_m input
function w_tires_radps = fcn(v_x_mps, dPsi_radps, r_tires_m, ...
            track_f_m, track_r_m, wb_f_m, wb_total_m)

w_tires_radps = WheelRotVelocities(v_x_mps, dPsi_radps, r_tires_m, ...
            track_f_m, track_r_m, wb_f_m, wb_total_m);

== matlab function Powertrain/Combustion Engine/Gearbox/TransmissionTorque ==
  data: T_clutch_Nm input; gear input; T_transmission_Nm output; i_gearset input
function T_transmission_Nm = fcn(T_clutch_Nm, gear, i_gearset)

T_transmission_Nm = TransmissionTorque(T_clutch_Nm, gear, i_gearset);

== matlab function Powertrain/Combustion Engine/GearSelection/enable_AutomaticGearbox/GearSelect ==
  data: drive_request input; gear_in input; gear output; w_engine_radps input; n_ub_rpm input; i_gearset input; shift_delay input; shift_request output
function [gear, shift_request] = fcn(drive_request, gear_in, ...
                            w_engine_radps, n_ub_rpm, i_gearset, shift_delay)

[gear, shift_request] = AutomaticGearbox(drive_request, gear_in, ...
                            w_engine_radps, n_ub_rpm, i_gearset, shift_delay);

== matlab function Powertrain/Combustion Engine/GearSelection/enable_ManualGearbox/ManualGearbox ==
  data: gear_in input; gear_desired input; gear output; w_engine_radps input; i_gearset input; shift_delay input; shift_request output
function [gear, shift_request] = fcn(gear_in, gear_desired, ...
                            w_engine_radps, i_gearset, shift_delay)

[gear, shift_request] = ManualGearbox(gear_in, gear_desired, ...
                            w_engine_radps, i_gearset, shift_delay);

== matlab function Powertrain/Combustion Engine/Clutch/ClutchTorque ==
  data: T_engine_Nm input; delta_rpm output; w_engine_in_radps input; w_transmission_radps input; wdot_transmission_radps2 input; gear input; T_max_cap_Nm input; T_cap_Nm output; T_loss_Nm output; T_clutch_Nm output; I_drivetrain_kgm2 input; clutch_act input
function [delta_rpm, T_cap_Nm, T_loss_Nm, T_clutch_Nm] = fcn(T_engine_Nm, ...
                              w_engine_in_radps, w_transmission_radps, ...
                              wdot_transmission_radps2, gear, T_max_cap_Nm, ...
                              I_drivetrain_kgm2, clutch_act)

[delta_rpm, T_cap_Nm, T_loss_Nm, T_clutch_Nm] = ClutchTorque(T_engine_Nm, ...
                              w_engine_in_radps, w_transmission_radps, ...
                              wdot_transmission_radps2, gear, T_max_cap_Nm, ...
                              I_drivetrain_kgm2, clutch_act);

== matlab function Powertrain/Combustion Engine/Clutch/EngineDynamics ==
  data: T_engine_Nm input; I_engine_kgm2 input; I_output_kgm2 input; delta_rpm input; wdot_engine_radps2 output; T_cap_Nm input
function wdot_engine_radps2 = fcn(T_engine_Nm, I_engine_kgm2, ...
                              I_output_kgm2, delta_rpm, T_cap_Nm)

wdot_engine_radps2 = EngineDynamics(T_engine_Nm, I_engine_kgm2, ...
                              I_output_kgm2, delta_rpm, T_cap_Nm);

== matlab function Powertrain/Combustion Engine/Engine/enable_ThrottleInterface/EngineLimiter ==
  data: p_throttle_desired_pos input; cutoff output; n_limiter_rpm input; n_engine_rpm input
function cutoff = fcn(p_throttle_desired_pos, n_limiter_rpm, n_engine_rpm)

cutoff = EngineLimiter(p_throttle_desired_pos, n_limiter_rpm, n_engine_rpm);

== matlab function Powertrain/Combustion Engine/Engine/enable_ThrottleInterface/IdleSpeedControl ==
  data: n_idle_rpm input; idle_control output; n_engine_rpm input
function idle_control = fcn(n_idle_rpm, n_engine_rpm)

idle_control = IdleSpeedControl(n_idle_rpm, n_engine_rpm);

== matlab function Powertrain/Combustion Engine/Engine/enable_ForceInterface/EngineLimiter ==
  data: F_x_request_N input; cutoff output; n_limiter_rpm input; n_engine_rpm input
function cutoff = fcn(F_x_request_N, n_limiter_rpm, n_engine_rpm)

cutoff = EngineLimiter(F_x_request_N, n_limiter_rpm, n_engine_rpm);

== matlab function Powertrain/Combustion Engine/Engine/enable_ForceInterface/ForceRequestConverter ==
  data: F_x_request_N input; T_request_Nm output; tire_radius_m input; i_c input; i_f input; i_r input; i_gearset input; p_torque_rear input; gear_in input
function T_request_Nm = fcn(F_x_request_N, tire_radius_m, i_c, i_f, i_r, i_gearset, p_torque_rear, gear_in)

T_request_Nm = ForceRequestConverter(F_x_request_N, tire_radius_m, i_c, i_f, i_r, i_gearset, p_torque_rear, gear_in);

== matlab function Powertrain/Combustion Engine/Engine/enable_ForceInterface/IdleSpeedControl ==
  data: n_idle_rpm input; idle_control output; n_engine_rpm input
function idle_control = fcn(n_idle_rpm, n_engine_rpm)

idle_control = IdleSpeedControl(n_idle_rpm, n_engine_rpm);

== matlab function Powertrain/Combustion Engine/Engine/enable_ForceInterface/ThrottleRequest ==
  data: T_request_Nm input; T_engine_Nm output; T_max_Nm input; T_min_Nm input; p_throttle_pos output
function [T_engine_Nm, p_throttle_pos] = fcn(T_request_Nm, T_max_Nm, T_min_Nm)

[T_engine_Nm, p_throttle_pos] = ThrottleRequest(T_request_Nm, T_max_Nm, T_min_Nm);

== matlab function Powertrain/Combustion Engine/Gearbox/TransmissionVelocity ==
  data: i_gearset input; w_transmission_radps output; gear input; w_diff_radps input
function w_transmission_radps = fcn(i_gearset, gear, w_diff_radps)

w_transmission_radps = TransmissionVelocity(i_gearset, gear, w_diff_radps);
